simulink model "TST_HLSDem_SelectParameter"  (R2016b)
settings: Solver=FixedStepDiscrete  StartTime=0.0  StopTime=simTime  FixedStep=sampleTime  RelTol=1e-3
values from neighbouring files (symbols this model uses):
  testCase = 1    [initTST_HLSDem_SelectParameter_001.m]    (also in initTST_HLSDem_SelectParameter_002.m = 2; initTST_HLSDem_SelectParameter_003.m = 3; initTST_HLSDem_SelectParameter_004.m = 4; initTST_HLSDem_SelectParameter_005.m = 5)
libraries: simulink x146, UnitTest_Lib x140
(part 4 of 4)

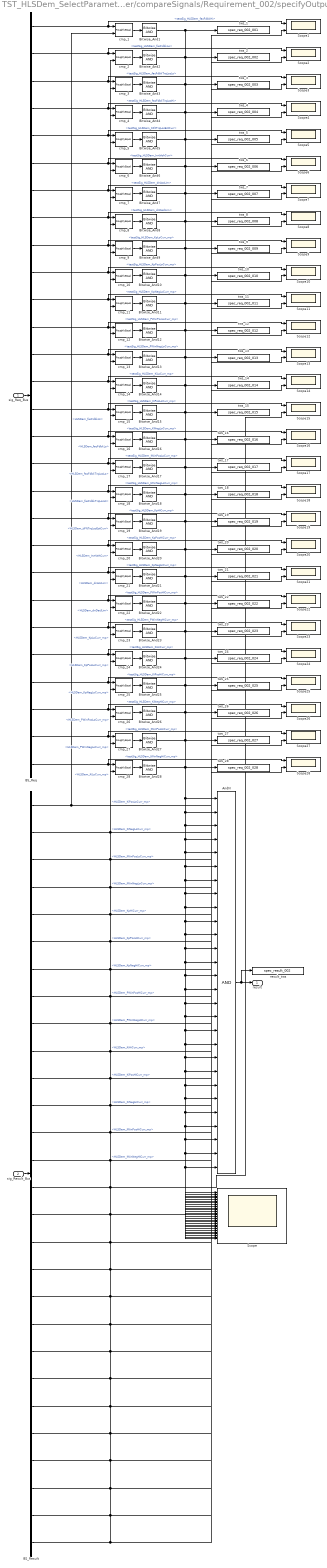
== system TST_HLSDem_SelectParameter/compareSignals/Requirement_002/specifyOutputs ==
  sig_Req_Bus : Inport
  sig_Result_Bus : Inport  Port=2
  AndN : Logic  Inputs=28
  BS_Req : BusSelector  OutputSignals=testSig_HLSDem_facFdbkHi,testSig_HLSDem_facFdbkLo,testSig_HLSDem_facFdbkTrqLosLo,testSig_HLSDem_facFdbkTrqLosHi,testSig_HLSDem_tiFltTrqLosEstCurr,testSig_HLSDem_InrtVehCurr,testSig_HLSDem_dnAccLim,testSig_HLSDem_dnDeclLim,testSig_HLSDem_KpLoCurr_mp,testSig_HLSDem_KpPosLoCurr_mp,testSig_HLSDem_KpNegLoCurr_mp,testSig_HLSDem_PWinPosLoCurr_mp,testSig_HLSDem_PWinNegLoCurr_mp,testSig_HLSDem_KiLoCurr_mp,testSig_HLSDem_KiPosLoCurr_mp,testSig_HLSDem_KiNegLoCurr_mp,testSig_HLSDem_IWinPosLoCurr_mp,testSig_HLSDem_IWinNegLoCurr_mp,testSig_HLSDem_KpHiCurr_mp,testSig_HLSDem_KpPosHiCurr_mp,testSig_HLSDem_KpNegHiCurr_mp,testSig_HLSDem_PWinPosHiCurr_mp,testSig_HLSDem_PWinNegHiCurr_mp,testSig_HLSDem_KiHiCurr_mp,testSig_HLSDem_KiPosHiCurr_mp,testSig_HLSDem_KiNegHiCurr_mp,testSig_HLSDem_IWinPosHiCurr_mp,testSig_HLSDem_IWinNegHiCurr_mp
  BS_Result : BusSelector  OutputSignals=HLSDem_facFdbkHi,HLSDem_facFdbkLo,HLSDem_facFdbkTrqLosLo,HLSDem_facFdbkTrqLosHi,HLSDem_tiFltTrqLosEstCurr,HLSDem_InrtVehCurr,HLSDem_dnAccLim,HLSDem_dnDeclLim,HLSDem_KpLoCurr_mp,HLSDem_KpPosLoCurr_mp,HLSDem_KpNegLoCurr_mp,HLSDem_PWinPosLoCurr_mp,HLSDem_PWinNegLoCurr_mp,HLSDem_KiLoCurr_mp,HLSDem_KiPosLoCurr_mp,HLSDem_KiNegLoCurr_mp,HLSDem_IWinPosLoCurr_mp,HLSDem_IWinNegLoCurr_mp,HLSDem_KpHiCurr_mp,HLSDem_KpPosHiCurr_mp,HLSDem_KpNegHiCurr_mp,HLSDem_PWinPosHiCurr_mp,HLSDem_PWinNegHiCurr_mp,HLSDem_KiHiCurr_mp,HLSDem_KiPosHiCurr_mp,HLSDem_KiNegHiCurr_mp,HLSDem_IWinPosHiCurr_mp,HLSDem_IWinNegHiCurr_mp
  Bitwise_And{1..28} (28 alike) : simulink/Logic and Bit Operations/Bitwise Operator  logicop=AND  UseBitMask=off  BitMask=bin2dec('11011001')  BitMaskRealWorld=Stored Integer
  Scope : Scope  NumInputPorts=28
  Scope{1..28} (28 alike) : Scope  NumInputPorts=2
  cmp_{1..6,9..28} (26 alike) : UnitTest_Lib/RoughlyEqual  slope=0.1
  cmp_7 : UnitTest_Lib/RoughlyEqual  slope=10
  cmp_8 : UnitTest_Lib/RoughlyEqual  slope=10
  result_tws : ToWorkspace  VariableName=spec_result_002
  tws_1 : ToWorkspace  VariableName=spec_req_002_001
  tws_10 : ToWorkspace  VariableName=spec_req_002_010
  tws_11 : ToWorkspace  VariableName=spec_req_002_011
  tws_12 : ToWorkspace  VariableName=spec_req_002_012
  tws_13 : ToWorkspace  VariableName=spec_req_002_013
  tws_14 : ToWorkspace  VariableName=spec_req_002_014
  tws_15 : ToWorkspace  VariableName=spec_req_002_015
  tws_16 : ToWorkspace  VariableName=spec_req_002_016
  tws_17 : ToWorkspace  VariableName=spec_req_002_017
  tws_18 : ToWorkspace  VariableName=spec_req_002_018
  tws_19 : ToWorkspace  VariableName=spec_req_002_019
  tws_2 : ToWorkspace  VariableName=spec_req_002_002
  tws_20 : ToWorkspace  VariableName=spec_req_002_020
  tws_21 : ToWorkspace  VariableName=spec_req_002_021
  tws_22 : ToWorkspace  VariableName=spec_req_002_022
  tws_23 : ToWorkspace  VariableName=spec_req_002_023
  tws_24 : ToWorkspace  VariableName=spec_req_002_024
  tws_25 : ToWorkspace  VariableName=spec_req_002_025
  tws_26 : ToWorkspace  VariableName=spec_req_002_026
  tws_27 : ToWorkspace  VariableName=spec_req_002_027
  tws_28 : ToWorkspace  VariableName=spec_req_002_028
  tws_3 : ToWorkspace  VariableName=spec_req_002_003
  tws_4 : ToWorkspace  VariableName=spec_req_002_004
  tws_5 : ToWorkspace  VariableName=spec_req_002_005
  tws_6 : ToWorkspace  VariableName=spec_req_002_006
  tws_7 : ToWorkspace  VariableName=spec_req_002_007
  tws_8 : ToWorkspace  VariableName=spec_req_002_008
  tws_9 : ToWorkspace  VariableName=spec_req_002_009
  result : Outport
  wires:
  sig_Req_Bus/1 -> BS_Req/1
  sig_Result_Bus/1 -> BS_Result/1
  AndN/1 -> result/1, result_tws/1
  BS_Req/1 -> cmp_1/1, Scope1/1  "<testSig_HLSDem_facFdbkHi>"
  BS_Result/1 -> cmp_1/2, Scope1/2  "<HLSDem_facFdbkHi>"
  cmp_1/1 -> Bitwise_And1/1
  Bitwise_And1/1 -> AndN/1, Scope/1, tws_1/1
  BS_Req/2 -> cmp_2/1, Scope2/1  "<testSig_HLSDem_facFdbkLo>"
  BS_Result/2 -> cmp_2/2, Scope2/2  "<HLSDem_facFdbkLo>"
  cmp_2/1 -> Bitwise_And2/1
  Bitwise_And2/1 -> AndN/2, Scope/2, tws_2/1
  BS_Req/3 -> cmp_3/1, Scope3/1  "<testSig_HLSDem_facFdbkTrqLosLo>"
  BS_Result/3 -> cmp_3/2, Scope3/2  "<HLSDem_facFdbkTrqLosLo>"
  cmp_3/1 -> Bitwise_And3/1
  Bitwise_And3/1 -> AndN/3, Scope/3, tws_3/1
  BS_Req/4 -> cmp_4/1, Scope4/1  "<testSig_HLSDem_facFdbkTrqLosHi>"
  BS_Result/4 -> cmp_4/2, Scope4/2  "<HLSDem_facFdbkTrqLosHi>"
  cmp_4/1 -> Bitwise_And4/1
  Bitwise_And4/1 -> AndN/4, Scope/4, tws_4/1
  BS_Req/5 -> cmp_5/1, Scope5/1  "<testSig_HLSDem_tiFltTrqLosEstCurr>"
  BS_Result/5 -> cmp_5/2, Scope5/2  "<HLSDem_tiFltTrqLosEstCurr>"
  cmp_5/1 -> Bitwise_And5/1
  Bitwise_And5/1 -> AndN/5, Scope/5, tws_5/1
  BS_Req/6 -> cmp_6/1, Scope6/1  "<testSig_HLSDem_InrtVehCurr>"
  BS_Result/6 -> cmp_6/2, Scope6/2  "<HLSDem_InrtVehCurr>"
  cmp_6/1 -> Bitwise_And6/1
  Bitwise_And6/1 -> AndN/6, Scope/6, tws_6/1
  BS_Req/7 -> cmp_7/1, Scope7/1  "<testSig_HLSDem_dnAccLim>"
  BS_Result/7 -> cmp_7/2, Scope7/2  "<HLSDem_dnAccLim>"
  cmp_7/1 -> Bitwise_And7/1
  Bitwise_And7/1 -> AndN/7, Scope/7, tws_7/1
  BS_Req/8 -> cmp_8/1, Scope8/1  "<testSig_HLSDem_dnDeclLim>"
  BS_Result/8 -> cmp_8/2, Scope8/2  "<HLSDem_dnDeclLim>"
  cmp_8/1 -> Bitwise_And8/1
  Bitwise_And8/1 -> AndN/8, Scope/8, tws_8/1
  BS_Req/9 -> cmp_9/1, Scope9/1  "<testSig_HLSDem_KpLoCurr_mp>"
  BS_Result/9 -> cmp_9/2, Scope9/2  "<HLSDem_KpLoCurr_mp>"
  cmp_9/1 -> Bitwise_And9/1
  Bitwise_And9/1 -> AndN/9, Scope/9, tws_9/1
  BS_Req/10 -> cmp_10/1, Scope10/1  "<testSig_HLSDem_KpPosLoCurr_mp>"
  BS_Result/10 -> cmp_10/2, Scope10/2  "<HLSDem_KpPosLoCurr_mp>"
  cmp_10/1 -> Bitwise_And10/1
  Bitwise_And10/1 -> AndN/10, Scope/10, tws_10/1
  BS_Req/11 -> cmp_11/1, Scope11/1  "<testSig_HLSDem_KpNegLoCurr_mp>"
  BS_Result/11 -> cmp_11/2, Scope11/2  "<HLSDem_KpNegLoCurr_mp>"
  cmp_11/1 -> Bitwise_And11/1
  Bitwise_And11/1 -> AndN/11, Scope/11, tws_11/1
  BS_Req/12 -> cmp_12/1, Scope12/1  "<testSig_HLSDem_PWinPosLoCurr_mp>"
  BS_Result/12 -> cmp_12/2, Scope12/2  "<HLSDem_PWinPosLoCurr_mp>"
  cmp_12/1 -> Bitwise_And12/1
  Bitwise_And12/1 -> AndN/12, Scope/12, tws_12/1
  BS_Req/13 -> cmp_13/1, Scope13/1  "<testSig_HLSDem_PWinNegLoCurr_mp>"
  BS_Result/13 -> cmp_13/2, Scope13/2  "<HLSDem_PWinNegLoCurr_mp>"
  cmp_13/1 -> Bitwise_And13/1
  Bitwise_And13/1 -> AndN/13, Scope/13, tws_13/1
  BS_Req/14 -> cmp_14/1, Scope14/1  "<testSig_HLSDem_KiLoCurr_mp>"
  BS_Result/14 -> cmp_14/2, Scope14/2  "<HLSDem_KiLoCurr_mp>"
  cmp_14/1 -> Bitwise_And14/1
  Bitwise_And14/1 -> AndN/14, Scope/14, tws_14/1
  BS_Req/15 -> cmp_15/1, Scope15/1  "<testSig_HLSDem_KiPosLoCurr_mp>"
  BS_Result/15 -> cmp_15/2, Scope15/2  "<HLSDem_KiPosLoCurr_mp>"
  cmp_15/1 -> Bitwise_And15/1
  Bitwise_And15/1 -> AndN/15, Scope/15, tws_15/1
  BS_Req/16 -> cmp_16/1, Scope16/1  "<testSig_HLSDem_KiNegLoCurr_mp>"
  BS_Result/16 -> cmp_16/2, Scope16/2  "<HLSDem_KiNegLoCurr_mp>"
  cmp_16/1 -> Bitwise_And16/1
  Bitwise_And16/1 -> AndN/16, Scope/16, tws_16/1
  BS_Req/17 -> cmp_17/1, Scope17/1  "<testSig_HLSDem_IWinPosLoCurr_mp>"
  BS_Result/17 -> cmp_17/2, Scope17/2  "<HLSDem_IWinPosLoCurr_mp>"
  cmp_17/1 -> Bitwise_And17/1
  Bitwise_And17/1 -> AndN/17, Scope/17, tws_17/1
  BS_Req/18 -> cmp_18/1, Scope18/1  "<testSig_HLSDem_IWinNegLoCurr_mp>"
  BS_Result/18 -> cmp_18/2, Scope18/2  "<HLSDem_IWinNegLoCurr_mp>"
  cmp_18/1 -> Bitwise_And18/1
  Bitwise_And18/1 -> AndN/18, Scope/18, tws_18/1
  BS_Req/19 -> cmp_19/1, Scope19/1  "<testSig_HLSDem_KpHiCurr_mp>"
  BS_Result/19 -> cmp_19/2, Scope19/2  "<HLSDem_KpHiCurr_mp>"
  cmp_19/1 -> Bitwise_And19/1
  Bitwise_And19/1 -> AndN/19, Scope/19, tws_19/1
  BS_Req/20 -> cmp_20/1, Scope20/1  "<testSig_HLSDem_KpPosHiCurr_mp>"
  BS_Result/20 -> cmp_20/2, Scope20/2  "<HLSDem_KpPosHiCurr_mp>"
  cmp_20/1 -> Bitwise_And20/1
  Bitwise_And20/1 -> AndN/20, Scope/20, tws_20/1
  BS_Req/21 -> cmp_21/1, Scope21/1  "<testSig_HLSDem_KpNegHiCurr_mp>"
  BS_Result/21 -> cmp_21/2, Scope21/2  "<HLSDem_KpNegHiCurr_mp>"
  cmp_21/1 -> Bitwise_And21/1
  Bitwise_And21/1 -> AndN/21, Scope/21, tws_21/1
  BS_Req/22 -> cmp_22/1, Scope22/1  "<testSig_HLSDem_PWinPosHiCurr_mp>"
  BS_Result/22 -> cmp_22/2, Scope22/2  "<HLSDem_PWinPosHiCurr_mp>"
  cmp_22/1 -> Bitwise_And22/1
  Bitwise_And22/1 -> AndN/22, Scope/22, tws_22/1
  BS_Req/23 -> cmp_23/1, Scope23/1  "<testSig_HLSDem_PWinNegHiCurr_mp>"
  BS_Result/23 -> cmp_23/2, Scope23/2  "<HLSDem_PWinNegHiCurr_mp>"
  cmp_23/1 -> Bitwise_And23/1
  Bitwise_And23/1 -> AndN/23, Scope/23, tws_23/1
  BS_Req/24 -> cmp_24/1, Scope24/1  "<testSig_HLSDem_KiHiCurr_mp>"
  BS_Result/24 -> cmp_24/2, Scope24/2  "<HLSDem_KiHiCurr_mp>"
  cmp_24/1 -> Bitwise_And24/1
  Bitwise_And24/1 -> AndN/24, Scope/24, tws_24/1
  BS_Req/25 -> cmp_25/1, Scope25/1  "<testSig_HLSDem_KiPosHiCurr_mp>"
  BS_Result/25 -> cmp_25/2, Scope25/2  "<HLSDem_KiPosHiCurr_mp>"
  cmp_25/1 -> Bitwise_And25/1
  Bitwise_And25/1 -> AndN/25, Scope/25, tws_25/1
  BS_Req/26 -> cmp_26/1, Scope26/1  "<testSig_HLSDem_KiNegHiCurr_mp>"
  BS_Result/26 -> cmp_26/2, Scope26/2  "<HLSDem_KiNegHiCurr_mp>"
  cmp_26/1 -> Bitwise_And26/1
  Bitwise_And26/1 -> AndN/26, Scope/26, tws_26/1
  BS_Req/27 -> cmp_27/1, Scope27/1  "<testSig_HLSDem_IWinPosHiCurr_mp>"
  BS_Result/27 -> cmp_27/2, Scope27/2  "<HLSDem_IWinPosHiCurr_mp>"
  cmp_27/1 -> Bitwise_And27/1
  Bitwise_And27/1 -> AndN/27, Scope/27, tws_27/1
  BS_Req/28 -> cmp_28/1, Scope28/1  "<testSig_HLSDem_IWinNegHiCurr_mp>"
  BS_Result/28 -> cmp_28/2, Scope28/2  "<HLSDem_IWinNegHiCurr_mp>"
  cmp_28/1 -> Bitwise_And28/1
  Bitwise_And28/1 -> AndN/28, Scope/28, tws_28/1

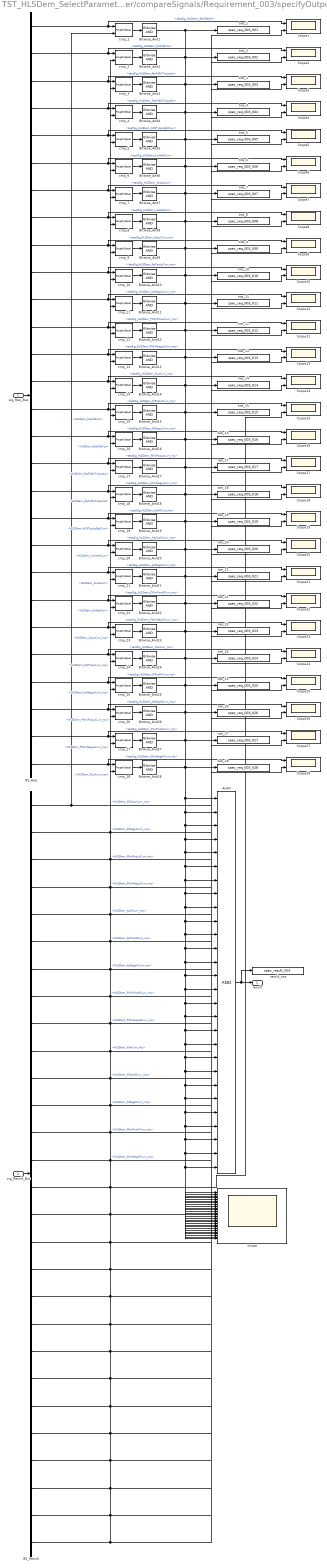
== system TST_HLSDem_SelectParameter/compareSignals/Requirement_003/specifyOutputs ==
  sig_Req_Bus : Inport
  sig_Result_Bus : Inport  Port=2
  AndN : Logic  Inputs=28
  BS_Req : BusSelector  OutputSignals=testSig_HLSDem_facFdbkHi,testSig_HLSDem_facFdbkLo,testSig_HLSDem_facFdbkTrqLosLo,testSig_HLSDem_facFdbkTrqLosHi,testSig_HLSDem_tiFltTrqLosEstCurr,testSig_HLSDem_InrtVehCurr,testSig_HLSDem_dnAccLim,testSig_HLSDem_dnDeclLim,testSig_HLSDem_KpLoCurr_mp,testSig_HLSDem_KpPosLoCurr_mp,testSig_HLSDem_KpNegLoCurr_mp,testSig_HLSDem_PWinPosLoCurr_mp,testSig_HLSDem_PWinNegLoCurr_mp,testSig_HLSDem_KiLoCurr_mp,testSig_HLSDem_KiPosLoCurr_mp,testSig_HLSDem_KiNegLoCurr_mp,testSig_HLSDem_IWinPosLoCurr_mp,testSig_HLSDem_IWinNegLoCurr_mp,testSig_HLSDem_KpHiCurr_mp,testSig_HLSDem_KpPosHiCurr_mp,testSig_HLSDem_KpNegHiCurr_mp,testSig_HLSDem_PWinPosHiCurr_mp,testSig_HLSDem_PWinNegHiCurr_mp,testSig_HLSDem_KiHiCurr_mp,testSig_HLSDem_KiPosHiCurr_mp,testSig_HLSDem_KiNegHiCurr_mp,testSig_HLSDem_IWinPosHiCurr_mp,testSig_HLSDem_IWinNegHiCurr_mp
  BS_Result : BusSelector  OutputSignals=HLSDem_facFdbkHi,HLSDem_facFdbkLo,HLSDem_facFdbkTrqLosLo,HLSDem_facFdbkTrqLosHi,HLSDem_tiFltTrqLosEstCurr,HLSDem_InrtVehCurr,HLSDem_dnAccLim,HLSDem_dnDeclLim,HLSDem_KpLoCurr_mp,HLSDem_KpPosLoCurr_mp,HLSDem_KpNegLoCurr_mp,HLSDem_PWinPosLoCurr_mp,HLSDem_PWinNegLoCurr_mp,HLSDem_KiLoCurr_mp,HLSDem_KiPosLoCurr_mp,HLSDem_KiNegLoCurr_mp,HLSDem_IWinPosLoCurr_mp,HLSDem_IWinNegLoCurr_mp,HLSDem_KpHiCurr_mp,HLSDem_KpPosHiCurr_mp,HLSDem_KpNegHiCurr_mp,HLSDem_PWinPosHiCurr_mp,HLSDem_PWinNegHiCurr_mp,HLSDem_KiHiCurr_mp,HLSDem_KiPosHiCurr_mp,HLSDem_KiNegHiCurr_mp,HLSDem_IWinPosHiCurr_mp,HLSDem_IWinNegHiCurr_mp
  Bitwise_And{1..28} (28 alike) : simulink/Logic and Bit Operations/Bitwise Operator  logicop=AND  UseBitMask=off  BitMask=bin2dec('11011001')  BitMaskRealWorld=Stored Integer
  Scope : Scope  NumInputPorts=28
  Scope{1..28} (28 alike) : Scope  NumInputPorts=2
  cmp_{1..6,9..28} (26 alike) : UnitTest_Lib/RoughlyEqual  slope=0.1
  cmp_7 : UnitTest_Lib/RoughlyEqual  slope=1
  cmp_8 : UnitTest_Lib/RoughlyEqual  slope=1
  result_tws : ToWorkspace  VariableName=spec_result_003
  tws_1 : ToWorkspace  VariableName=spec_req_003_001
  tws_10 : ToWorkspace  VariableName=spec_req_003_010
  tws_11 : ToWorkspace  VariableName=spec_req_003_011
  tws_12 : ToWorkspace  VariableName=spec_req_003_012
  tws_13 : ToWorkspace  VariableName=spec_req_003_013
  tws_14 : ToWorkspace  VariableName=spec_req_003_014
  tws_15 : ToWorkspace  VariableName=spec_req_003_015
  tws_16 : ToWorkspace  VariableName=spec_req_003_016
  tws_17 : ToWorkspace  VariableName=spec_req_003_017
  tws_18 : ToWorkspace  VariableName=spec_req_003_018
  tws_19 : ToWorkspace  VariableName=spec_req_003_019
  tws_2 : ToWorkspace  VariableName=spec_req_003_002
  tws_20 : ToWorkspace  VariableName=spec_req_003_020
  tws_21 : ToWorkspace  VariableName=spec_req_003_021
  tws_22 : ToWorkspace  VariableName=spec_req_003_022
  tws_23 : ToWorkspace  VariableName=spec_req_003_023
  tws_24 : ToWorkspace  VariableName=spec_req_003_024
  tws_25 : ToWorkspace  VariableName=spec_req_003_025
  tws_26 : ToWorkspace  VariableName=spec_req_003_026
  tws_27 : ToWorkspace  VariableName=spec_req_003_027
  tws_28 : ToWorkspace  VariableName=spec_req_003_028
  tws_3 : ToWorkspace  VariableName=spec_req_003_003
  tws_4 : ToWorkspace  VariableName=spec_req_003_004
  tws_5 : ToWorkspace  VariableName=spec_req_003_005
  tws_6 : ToWorkspace  VariableName=spec_req_003_006
  tws_7 : ToWorkspace  VariableName=spec_req_003_007
  tws_8 : ToWorkspace  VariableName=spec_req_003_008
  tws_9 : ToWorkspace  VariableName=spec_req_003_009
  result : Outport
  wires:
  sig_Req_Bus/1 -> BS_Req/1
  sig_Result_Bus/1 -> BS_Result/1
  AndN/1 -> result/1, result_tws/1
  BS_Req/1 -> cmp_1/1, Scope1/1  "<testSig_HLSDem_facFdbkHi>"
  BS_Result/1 -> cmp_1/2, Scope1/2  "<HLSDem_facFdbkHi>"
  cmp_1/1 -> Bitwise_And1/1
  Bitwise_And1/1 -> AndN/1, Scope/1, tws_1/1
  BS_Req/2 -> cmp_2/1, Scope2/1  "<testSig_HLSDem_facFdbkLo>"
  BS_Result/2 -> cmp_2/2, Scope2/2  "<HLSDem_facFdbkLo>"
  cmp_2/1 -> Bitwise_And2/1
  Bitwise_And2/1 -> AndN/2, Scope/2, tws_2/1
  BS_Req/3 -> cmp_3/1, Scope3/1  "<testSig_HLSDem_facFdbkTrqLosLo>"
  BS_Result/3 -> cmp_3/2, Scope3/2  "<HLSDem_facFdbkTrqLosLo>"
  cmp_3/1 -> Bitwise_And3/1
  Bitwise_And3/1 -> AndN/3, Scope/3, tws_3/1
  BS_Req/4 -> cmp_4/1, Scope4/1  "<testSig_HLSDem_facFdbkTrqLosHi>"
  BS_Result/4 -> cmp_4/2, Scope4/2  "<HLSDem_facFdbkTrqLosHi>"
  cmp_4/1 -> Bitwise_And4/1
  Bitwise_And4/1 -> AndN/4, Scope/4, tws_4/1
  BS_Req/5 -> cmp_5/1, Scope5/1  "<testSig_HLSDem_tiFltTrqLosEstCurr>"
  BS_Result/5 -> cmp_5/2, Scope5/2  "<HLSDem_tiFltTrqLosEstCurr>"
  cmp_5/1 -> Bitwise_And5/1
  Bitwise_And5/1 -> AndN/5, Scope/5, tws_5/1
  BS_Req/6 -> cmp_6/1, Scope6/1  "<testSig_HLSDem_InrtVehCurr>"
  BS_Result/6 -> cmp_6/2, Scope6/2  "<HLSDem_InrtVehCurr>"
  cmp_6/1 -> Bitwise_And6/1
  Bitwise_And6/1 -> AndN/6, Scope/6, tws_6/1
  BS_Req/7 -> cmp_7/1, Scope7/1  "<testSig_HLSDem_dnAccLim>"
  BS_Result/7 -> cmp_7/2, Scope7/2  "<HLSDem_dnAccLim>"
  cmp_7/1 -> Bitwise_And7/1
  Bitwise_And7/1 -> AndN/7, Scope/7, tws_7/1
  BS_Req/8 -> cmp_8/1, Scope8/1  "<testSig_HLSDem_dnDeclLim>"
  BS_Result/8 -> cmp_8/2, Scope8/2  "<HLSDem_dnDeclLim>"
  cmp_8/1 -> Bitwise_And8/1
  Bitwise_And8/1 -> AndN/8, Scope/8, tws_8/1
  BS_Req/9 -> cmp_9/1, Scope9/1  "<testSig_HLSDem_KpLoCurr_mp>"
  BS_Result/9 -> cmp_9/2, Scope9/2  "<HLSDem_KpLoCurr_mp>"
  cmp_9/1 -> Bitwise_And9/1
  Bitwise_And9/1 -> AndN/9, Scope/9, tws_9/1
  BS_Req/10 -> cmp_10/1, Scope10/1  "<testSig_HLSDem_KpPosLoCurr_mp>"
  BS_Result/10 -> cmp_10/2, Scope10/2  "<HLSDem_KpPosLoCurr_mp>"
  cmp_10/1 -> Bitwise_And10/1
  Bitwise_And10/1 -> AndN/10, Scope/10, tws_10/1
  BS_Req/11 -> cmp_11/1, Scope11/1  "<testSig_HLSDem_KpNegLoCurr_mp>"
  BS_Result/11 -> cmp_11/2, Scope11/2  "<HLSDem_KpNegLoCurr_mp>"
  cmp_11/1 -> Bitwise_And11/1
  Bitwise_And11/1 -> AndN/11, Scope/11, tws_11/1
  BS_Req/12 -> cmp_12/1, Scope12/1  "<testSig_HLSDem_PWinPosLoCurr_mp>"
  BS_Result/12 -> cmp_12/2, Scope12/2  "<HLSDem_PWinPosLoCurr_mp>"
  cmp_12/1 -> Bitwise_And12/1
  Bitwise_And12/1 -> AndN/12, Scope/12, tws_12/1
  BS_Req/13 -> cmp_13/1, Scope13/1  "<testSig_HLSDem_PWinNegLoCurr_mp>"
  BS_Result/13 -> cmp_13/2, Scope13/2  "<HLSDem_PWinNegLoCurr_mp>"
  cmp_13/1 -> Bitwise_And13/1
  Bitwise_And13/1 -> AndN/13, Scope/13, tws_13/1
  BS_Req/14 -> cmp_14/1, Scope14/1  "<testSig_HLSDem_KiLoCurr_mp>"
  BS_Result/14 -> cmp_14/2, Scope14/2  "<HLSDem_KiLoCurr_mp>"
  cmp_14/1 -> Bitwise_And14/1
  Bitwise_And14/1 -> AndN/14, Scope/14, tws_14/1
  BS_Req/15 -> cmp_15/1, Scope15/1  "<testSig_HLSDem_KiPosLoCurr_mp>"
  BS_Result/15 -> cmp_15/2, Scope15/2  "<HLSDem_KiPosLoCurr_mp>"
  cmp_15/1 -> Bitwise_And15/1
  Bitwise_And15/1 -> AndN/15, Scope/15, tws_15/1
  BS_Req/16 -> cmp_16/1, Scope16/1  "<testSig_HLSDem_KiNegLoCurr_mp>"
  BS_Result/16 -> cmp_16/2, Scope16/2  "<HLSDem_KiNegLoCurr_mp>"
  cmp_16/1 -> Bitwise_And16/1
  Bitwise_And16/1 -> AndN/16, Scope/16, tws_16/1
  BS_Req/17 -> cmp_17/1, Scope17/1  "<testSig_HLSDem_IWinPosLoCurr_mp>"
  BS_Result/17 -> cmp_17/2, Scope17/2  "<HLSDem_IWinPosLoCurr_mp>"
  cmp_17/1 -> Bitwise_And17/1
  Bitwise_And17/1 -> AndN/17, Scope/17, tws_17/1
  BS_Req/18 -> cmp_18/1, Scope18/1  "<testSig_HLSDem_IWinNegLoCurr_mp>"
  BS_Result/18 -> cmp_18/2, Scope18/2  "<HLSDem_IWinNegLoCurr_mp>"
  cmp_18/1 -> Bitwise_And18/1
  Bitwise_And18/1 -> AndN/18, Scope/18, tws_18/1
  BS_Req/19 -> cmp_19/1, Scope19/1  "<testSig_HLSDem_KpHiCurr_mp>"
  BS_Result/19 -> cmp_19/2, Scope19/2  "<HLSDem_KpHiCurr_mp>"
  cmp_19/1 -> Bitwise_And19/1
  Bitwise_And19/1 -> AndN/19, Scope/19, tws_19/1
  BS_Req/20 -> cmp_20/1, Scope20/1  "<testSig_HLSDem_KpPosHiCurr_mp>"
  BS_Result/20 -> cmp_20/2, Scope20/2  "<HLSDem_KpPosHiCurr_mp>"
  cmp_20/1 -> Bitwise_And20/1
  Bitwise_And20/1 -> AndN/20, Scope/20, tws_20/1
  BS_Req/21 -> cmp_21/1, Scope21/1  "<testSig_HLSDem_KpNegHiCurr_mp>"
  BS_Result/21 -> cmp_21/2, Scope21/2  "<HLSDem_KpNegHiCurr_mp>"
  cmp_21/1 -> Bitwise_And21/1
  Bitwise_And21/1 -> AndN/21, Scope/21, tws_21/1
  BS_Req/22 -> cmp_22/1, Scope22/1  "<testSig_HLSDem_PWinPosHiCurr_mp>"
  BS_Result/22 -> cmp_22/2, Scope22/2  "<HLSDem_PWinPosHiCurr_mp>"
  cmp_22/1 -> Bitwise_And22/1
  Bitwise_And22/1 -> AndN/22, Scope/22, tws_22/1
  BS_Req/23 -> cmp_23/1, Scope23/1  "<testSig_HLSDem_PWinNegHiCurr_mp>"
  BS_Result/23 -> cmp_23/2, Scope23/2  "<HLSDem_PWinNegHiCurr_mp>"
  cmp_23/1 -> Bitwise_And23/1
  Bitwise_And23/1 -> AndN/23, Scope/23, tws_23/1
  BS_Req/24 -> cmp_24/1, Scope24/1  "<testSig_HLSDem_KiHiCurr_mp>"
  BS_Result/24 -> cmp_24/2, Scope24/2  "<HLSDem_KiHiCurr_mp>"
  cmp_24/1 -> Bitwise_And24/1
  Bitwise_And24/1 -> AndN/24, Scope/24, tws_24/1
  BS_Req/25 -> cmp_25/1, Scope25/1  "<testSig_HLSDem_KiPosHiCurr_mp>"
  BS_Result/25 -> cmp_25/2, Scope25/2  "<HLSDem_KiPosHiCurr_mp>"
  cmp_25/1 -> Bitwise_And25/1
  Bitwise_And25/1 -> AndN/25, Scope/25, tws_25/1
  BS_Req/26 -> cmp_26/1, Scope26/1  "<testSig_HLSDem_KiNegHiCurr_mp>"
  BS_Result/26 -> cmp_26/2, Scope26/2  "<HLSDem_KiNegHiCurr_mp>"
  cmp_26/1 -> Bitwise_And26/1
  Bitwise_And26/1 -> AndN/26, Scope/26, tws_26/1
  BS_Req/27 -> cmp_27/1, Scope27/1  "<testSig_HLSDem_IWinPosHiCurr_mp>"
  BS_Result/27 -> cmp_27/2, Scope27/2  "<HLSDem_IWinPosHiCurr_mp>"
  cmp_27/1 -> Bitwise_And27/1
  Bitwise_And27/1 -> AndN/27, Scope/27, tws_27/1
  BS_Req/28 -> cmp_28/1, Scope28/1  "<testSig_HLSDem_IWinNegHiCurr_mp>"
  BS_Result/28 -> cmp_28/2, Scope28/2  "<HLSDem_IWinNegHiCurr_mp>"
  cmp_28/1 -> Bitwise_And28/1
  Bitwise_And28/1 -> AndN/28, Scope/28, tws_28/1

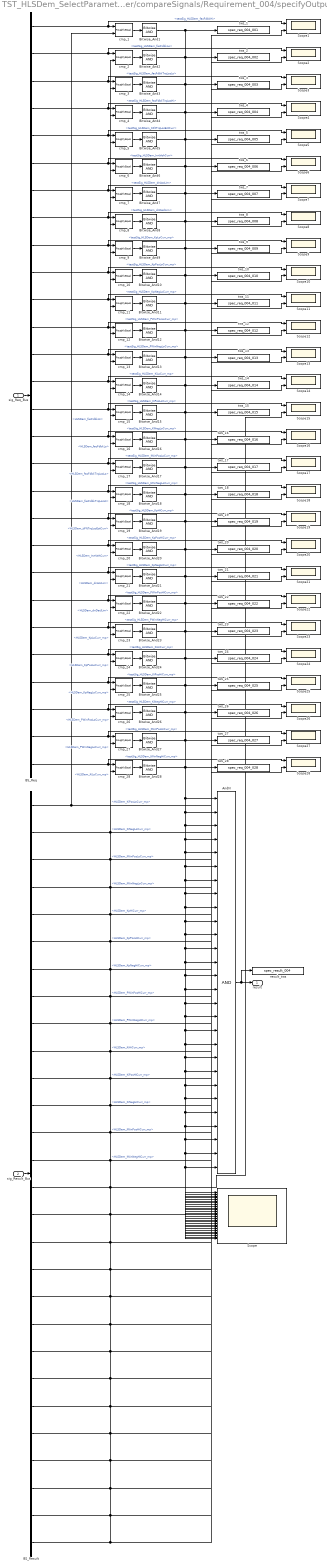
== system TST_HLSDem_SelectParameter/compareSignals/Requirement_004/specifyOutputs ==
  sig_Req_Bus : Inport
  sig_Result_Bus : Inport  Port=2
  AndN : Logic  Inputs=28
  BS_Req : BusSelector  OutputSignals=testSig_HLSDem_facFdbkHi,testSig_HLSDem_facFdbkLo,testSig_HLSDem_facFdbkTrqLosLo,testSig_HLSDem_facFdbkTrqLosHi,testSig_HLSDem_tiFltTrqLosEstCurr,testSig_HLSDem_InrtVehCurr,testSig_HLSDem_dnAccLim,testSig_HLSDem_dnDeclLim,testSig_HLSDem_KpLoCurr_mp,testSig_HLSDem_KpPosLoCurr_mp,testSig_HLSDem_KpNegLoCurr_mp,testSig_HLSDem_PWinPosLoCurr_mp,testSig_HLSDem_PWinNegLoCurr_mp,testSig_HLSDem_KiLoCurr_mp,testSig_HLSDem_KiPosLoCurr_mp,testSig_HLSDem_KiNegLoCurr_mp,testSig_HLSDem_IWinPosLoCurr_mp,testSig_HLSDem_IWinNegLoCurr_mp,testSig_HLSDem_KpHiCurr_mp,testSig_HLSDem_KpPosHiCurr_mp,testSig_HLSDem_KpNegHiCurr_mp,testSig_HLSDem_PWinPosHiCurr_mp,testSig_HLSDem_PWinNegHiCurr_mp,testSig_HLSDem_KiHiCurr_mp,testSig_HLSDem_KiPosHiCurr_mp,testSig_HLSDem_KiNegHiCurr_mp,testSig_HLSDem_IWinPosHiCurr_mp,testSig_HLSDem_IWinNegHiCurr_mp
  BS_Result : BusSelector  OutputSignals=HLSDem_facFdbkHi,HLSDem_facFdbkLo,HLSDem_facFdbkTrqLosLo,HLSDem_facFdbkTrqLosHi,HLSDem_tiFltTrqLosEstCurr,HLSDem_InrtVehCurr,HLSDem_dnAccLim,HLSDem_dnDeclLim,HLSDem_KpLoCurr_mp,HLSDem_KpPosLoCurr_mp,HLSDem_KpNegLoCurr_mp,HLSDem_PWinPosLoCurr_mp,HLSDem_PWinNegLoCurr_mp,HLSDem_KiLoCurr_mp,HLSDem_KiPosLoCurr_mp,HLSDem_KiNegLoCurr_mp,HLSDem_IWinPosLoCurr_mp,HLSDem_IWinNegLoCurr_mp,HLSDem_KpHiCurr_mp,HLSDem_KpPosHiCurr_mp,HLSDem_KpNegHiCurr_mp,HLSDem_PWinPosHiCurr_mp,HLSDem_PWinNegHiCurr_mp,HLSDem_KiHiCurr_mp,HLSDem_KiPosHiCurr_mp,HLSDem_KiNegHiCurr_mp,HLSDem_IWinPosHiCurr_mp,HLSDem_IWinNegHiCurr_mp
  Bitwise_And{1..28} (28 alike) : simulink/Logic and Bit Operations/Bitwise Operator  logicop=AND  UseBitMask=off  BitMask=bin2dec('11011001')  BitMaskRealWorld=Stored Integer
  Scope : Scope  NumInputPorts=28
  Scope{1..28} (28 alike) : Scope  NumInputPorts=2
  cmp_{1..6,9..28} (26 alike) : UnitTest_Lib/RoughlyEqual  slope=0.1
  cmp_7 : UnitTest_Lib/RoughlyEqual  slope=1
  cmp_8 : UnitTest_Lib/RoughlyEqual  slope=1
  result_tws : ToWorkspace  VariableName=spec_result_004
  tws_1 : ToWorkspace  VariableName=spec_req_004_001
  tws_10 : ToWorkspace  VariableName=spec_req_004_010
  tws_11 : ToWorkspace  VariableName=spec_req_004_011
  tws_12 : ToWorkspace  VariableName=spec_req_004_012
  tws_13 : ToWorkspace  VariableName=spec_req_004_013
  tws_14 : ToWorkspace  VariableName=spec_req_004_014
  tws_15 : ToWorkspace  VariableName=spec_req_004_015
  tws_16 : ToWorkspace  VariableName=spec_req_004_016
  tws_17 : ToWorkspace  VariableName=spec_req_004_017
  tws_18 : ToWorkspace  VariableName=spec_req_004_018
  tws_19 : ToWorkspace  VariableName=spec_req_004_019
  tws_2 : ToWorkspace  VariableName=spec_req_004_002
  tws_20 : ToWorkspace  VariableName=spec_req_004_020
  tws_21 : ToWorkspace  VariableName=spec_req_004_021
  tws_22 : ToWorkspace  VariableName=spec_req_004_022
  tws_23 : ToWorkspace  VariableName=spec_req_004_023
  tws_24 : ToWorkspace  VariableName=spec_req_004_024
  tws_25 : ToWorkspace  VariableName=spec_req_004_025
  tws_26 : ToWorkspace  VariableName=spec_req_004_026
  tws_27 : ToWorkspace  VariableName=spec_req_004_027
  tws_28 : ToWorkspace  VariableName=spec_req_004_028
  tws_3 : ToWorkspace  VariableName=spec_req_004_003
  tws_4 : ToWorkspace  VariableName=spec_req_004_004
  tws_5 : ToWorkspace  VariableName=spec_req_004_005
  tws_6 : ToWorkspace  VariableName=spec_req_004_006
  tws_7 : ToWorkspace  VariableName=spec_req_004_007
  tws_8 : ToWorkspace  VariableName=spec_req_004_008
  tws_9 : ToWorkspace  VariableName=spec_req_004_009
  result : Outport
  wires:
  sig_Req_Bus/1 -> BS_Req/1
  sig_Result_Bus/1 -> BS_Result/1
  AndN/1 -> result/1, result_tws/1
  BS_Req/1 -> cmp_1/1, Scope1/1  "<testSig_HLSDem_facFdbkHi>"
  BS_Result/1 -> cmp_1/2, Scope1/2  "<HLSDem_facFdbkHi>"
  cmp_1/1 -> Bitwise_And1/1
  Bitwise_And1/1 -> AndN/1, Scope/1, tws_1/1
  BS_Req/2 -> cmp_2/1, Scope2/1  "<testSig_HLSDem_facFdbkLo>"
  BS_Result/2 -> cmp_2/2, Scope2/2  "<HLSDem_facFdbkLo>"
  cmp_2/1 -> Bitwise_And2/1
  Bitwise_And2/1 -> AndN/2, Scope/2, tws_2/1
  BS_Req/3 -> cmp_3/1, Scope3/1  "<testSig_HLSDem_facFdbkTrqLosLo>"
  BS_Result/3 -> cmp_3/2, Scope3/2  "<HLSDem_facFdbkTrqLosLo>"
  cmp_3/1 -> Bitwise_And3/1
  Bitwise_And3/1 -> AndN/3, Scope/3, tws_3/1
  BS_Req/4 -> cmp_4/1, Scope4/1  "<testSig_HLSDem_facFdbkTrqLosHi>"
  BS_Result/4 -> cmp_4/2, Scope4/2  "<HLSDem_facFdbkTrqLosHi>"
  cmp_4/1 -> Bitwise_And4/1
  Bitwise_And4/1 -> AndN/4, Scope/4, tws_4/1
  BS_Req/5 -> cmp_5/1, Scope5/1  "<testSig_HLSDem_tiFltTrqLosEstCurr>"
  BS_Result/5 -> cmp_5/2, Scope5/2  "<HLSDem_tiFltTrqLosEstCurr>"
  cmp_5/1 -> Bitwise_And5/1
  Bitwise_And5/1 -> AndN/5, Scope/5, tws_5/1
  BS_Req/6 -> cmp_6/1, Scope6/1  "<testSig_HLSDem_InrtVehCurr>"
  BS_Result/6 -> cmp_6/2, Scope6/2  "<HLSDem_InrtVehCurr>"
  cmp_6/1 -> Bitwise_And6/1
  Bitwise_And6/1 -> AndN/6, Scope/6, tws_6/1
  BS_Req/7 -> cmp_7/1, Scope7/1  "<testSig_HLSDem_dnAccLim>"
  BS_Result/7 -> cmp_7/2, Scope7/2  "<HLSDem_dnAccLim>"
  cmp_7/1 -> Bitwise_And7/1
  Bitwise_And7/1 -> AndN/7, Scope/7, tws_7/1
  BS_Req/8 -> cmp_8/1, Scope8/1  "<testSig_HLSDem_dnDeclLim>"
  BS_Result/8 -> cmp_8/2, Scope8/2  "<HLSDem_dnDeclLim>"
  cmp_8/1 -> Bitwise_And8/1
  Bitwise_And8/1 -> AndN/8, Scope/8, tws_8/1
  BS_Req/9 -> cmp_9/1, Scope9/1  "<testSig_HLSDem_KpLoCurr_mp>"
  BS_Result/9 -> cmp_9/2, Scope9/2  "<HLSDem_KpLoCurr_mp>"
  cmp_9/1 -> Bitwise_And9/1
  Bitwise_And9/1 -> AndN/9, Scope/9, tws_9/1
  BS_Req/10 -> cmp_10/1, Scope10/1  "<testSig_HLSDem_KpPosLoCurr_mp>"
  BS_Result/10 -> cmp_10/2, Scope10/2  "<HLSDem_KpPosLoCurr_mp>"
  cmp_10/1 -> Bitwise_And10/1
  Bitwise_And10/1 -> AndN/10, Scope/10, tws_10/1
  BS_Req/11 -> cmp_11/1, Scope11/1  "<testSig_HLSDem_KpNegLoCurr_mp>"
  BS_Result/11 -> cmp_11/2, Scope11/2  "<HLSDem_KpNegLoCurr_mp>"
  cmp_11/1 -> Bitwise_And11/1
  Bitwise_And11/1 -> AndN/11, Scope/11, tws_11/1
  BS_Req/12 -> cmp_12/1, Scope12/1  "<testSig_HLSDem_PWinPosLoCurr_mp>"
  BS_Result/12 -> cmp_12/2, Scope12/2  "<HLSDem_PWinPosLoCurr_mp>"
  cmp_12/1 -> Bitwise_And12/1
  Bitwise_And12/1 -> AndN/12, Scope/12, tws_12/1
  BS_Req/13 -> cmp_13/1, Scope13/1  "<testSig_HLSDem_PWinNegLoCurr_mp>"
  BS_Result/13 -> cmp_13/2, Scope13/2  "<HLSDem_PWinNegLoCurr_mp>"
  cmp_13/1 -> Bitwise_And13/1
  Bitwise_And13/1 -> AndN/13, Scope/13, tws_13/1
  BS_Req/14 -> cmp_14/1, Scope14/1  "<testSig_HLSDem_KiLoCurr_mp>"
  BS_Result/14 -> cmp_14/2, Scope14/2  "<HLSDem_KiLoCurr_mp>"
  cmp_14/1 -> Bitwise_And14/1
  Bitwise_And14/1 -> AndN/14, Scope/14, tws_14/1
  BS_Req/15 -> cmp_15/1, Scope15/1  "<testSig_HLSDem_KiPosLoCurr_mp>"
  BS_Result/15 -> cmp_15/2, Scope15/2  "<HLSDem_KiPosLoCurr_mp>"
  cmp_15/1 -> Bitwise_And15/1
  Bitwise_And15/1 -> AndN/15, Scope/15, tws_15/1
  BS_Req/16 -> cmp_16/1, Scope16/1  "<testSig_HLSDem_KiNegLoCurr_mp>"
  BS_Result/16 -> cmp_16/2, Scope16/2  "<HLSDem_KiNegLoCurr_mp>"
  cmp_16/1 -> Bitwise_And16/1
  Bitwise_And16/1 -> AndN/16, Scope/16, tws_16/1
  BS_Req/17 -> cmp_17/1, Scope17/1  "<testSig_HLSDem_IWinPosLoCurr_mp>"
  BS_Result/17 -> cmp_17/2, Scope17/2  "<HLSDem_IWinPosLoCurr_mp>"
  cmp_17/1 -> Bitwise_And17/1
  Bitwise_And17/1 -> AndN/17, Scope/17, tws_17/1
  BS_Req/18 -> cmp_18/1, Scope18/1  "<testSig_HLSDem_IWinNegLoCurr_mp>"
  BS_Result/18 -> cmp_18/2, Scope18/2  "<HLSDem_IWinNegLoCurr_mp>"
  cmp_18/1 -> Bitwise_And18/1
  Bitwise_And18/1 -> AndN/18, Scope/18, tws_18/1
  BS_Req/19 -> cmp_19/1, Scope19/1  "<testSig_HLSDem_KpHiCurr_mp>"
  BS_Result/19 -> cmp_19/2, Scope19/2  "<HLSDem_KpHiCurr_mp>"
  cmp_19/1 -> Bitwise_And19/1
  Bitwise_And19/1 -> AndN/19, Scope/19, tws_19/1
  BS_Req/20 -> cmp_20/1, Scope20/1  "<testSig_HLSDem_KpPosHiCurr_mp>"
  BS_Result/20 -> cmp_20/2, Scope20/2  "<HLSDem_KpPosHiCurr_mp>"
  cmp_20/1 -> Bitwise_And20/1
  Bitwise_And20/1 -> AndN/20, Scope/20, tws_20/1
  BS_Req/21 -> cmp_21/1, Scope21/1  "<testSig_HLSDem_KpNegHiCurr_mp>"
  BS_Result/21 -> cmp_21/2, Scope21/2  "<HLSDem_KpNegHiCurr_mp>"
  cmp_21/1 -> Bitwise_And21/1
  Bitwise_And21/1 -> AndN/21, Scope/21, tws_21/1
  BS_Req/22 -> cmp_22/1, Scope22/1  "<testSig_HLSDem_PWinPosHiCurr_mp>"
  BS_Result/22 -> cmp_22/2, Scope22/2  "<HLSDem_PWinPosHiCurr_mp>"
  cmp_22/1 -> Bitwise_And22/1
  Bitwise_And22/1 -> AndN/22, Scope/22, tws_22/1
  BS_Req/23 -> cmp_23/1, Scope23/1  "<testSig_HLSDem_PWinNegHiCurr_mp>"
  BS_Result/23 -> cmp_23/2, Scope23/2  "<HLSDem_PWinNegHiCurr_mp>"
  cmp_23/1 -> Bitwise_And23/1
  Bitwise_And23/1 -> AndN/23, Scope/23, tws_23/1
  BS_Req/24 -> cmp_24/1, Scope24/1  "<testSig_HLSDem_KiHiCurr_mp>"
  BS_Result/24 -> cmp_24/2, Scope24/2  "<HLSDem_KiHiCurr_mp>"
  cmp_24/1 -> Bitwise_And24/1
  Bitwise_And24/1 -> AndN/24, Scope/24, tws_24/1
  BS_Req/25 -> cmp_25/1, Scope25/1  "<testSig_HLSDem_KiPosHiCurr_mp>"
  BS_Result/25 -> cmp_25/2, Scope25/2  "<HLSDem_KiPosHiCurr_mp>"
  cmp_25/1 -> Bitwise_And25/1
  Bitwise_And25/1 -> AndN/25, Scope/25, tws_25/1
  BS_Req/26 -> cmp_26/1, Scope26/1  "<testSig_HLSDem_KiNegHiCurr_mp>"
  BS_Result/26 -> cmp_26/2, Scope26/2  "<HLSDem_KiNegHiCurr_mp>"
  cmp_26/1 -> Bitwise_And26/1
  Bitwise_And26/1 -> AndN/26, Scope/26, tws_26/1
  BS_Req/27 -> cmp_27/1, Scope27/1  "<testSig_HLSDem_IWinPosHiCurr_mp>"
  BS_Result/27 -> cmp_27/2, Scope27/2  "<HLSDem_IWinPosHiCurr_mp>"
  cmp_27/1 -> Bitwise_And27/1
  Bitwise_And27/1 -> AndN/27, Scope/27, tws_27/1
  BS_Req/28 -> cmp_28/1, Scope28/1  "<testSig_HLSDem_IWinNegHiCurr_mp>"
  BS_Result/28 -> cmp_28/2, Scope28/2  "<HLSDem_IWinNegHiCurr_mp>"
  cmp_28/1 -> Bitwise_And28/1
  Bitwise_And28/1 -> AndN/28, Scope/28, tws_28/1

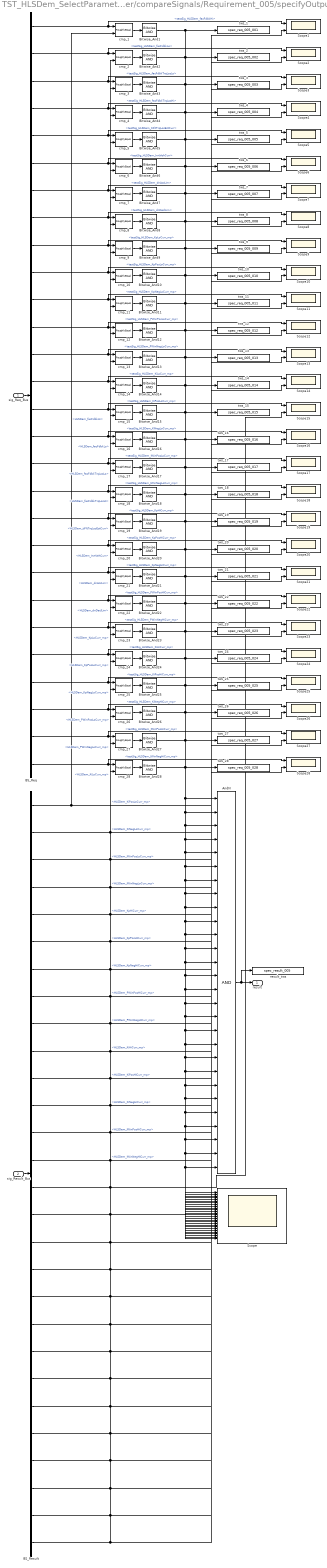
== system TST_HLSDem_SelectParameter/compareSignals/Requirement_005/specifyOutputs ==
  sig_Req_Bus : Inport
  sig_Result_Bus : Inport  Port=2
  AndN : Logic  Inputs=28
  BS_Req : BusSelector  OutputSignals=testSig_HLSDem_facFdbkHi,testSig_HLSDem_facFdbkLo,testSig_HLSDem_facFdbkTrqLosLo,testSig_HLSDem_facFdbkTrqLosHi,testSig_HLSDem_tiFltTrqLosEstCurr,testSig_HLSDem_InrtVehCurr,testSig_HLSDem_dnAccLim,testSig_HLSDem_dnDeclLim,testSig_HLSDem_KpLoCurr_mp,testSig_HLSDem_KpPosLoCurr_mp,testSig_HLSDem_KpNegLoCurr_mp,testSig_HLSDem_PWinPosLoCurr_mp,testSig_HLSDem_PWinNegLoCurr_mp,testSig_HLSDem_KiLoCurr_mp,testSig_HLSDem_KiPosLoCurr_mp,testSig_HLSDem_KiNegLoCurr_mp,testSig_HLSDem_IWinPosLoCurr_mp,testSig_HLSDem_IWinNegLoCurr_mp,testSig_HLSDem_KpHiCurr_mp,testSig_HLSDem_KpPosHiCurr_mp,testSig_HLSDem_KpNegHiCurr_mp,testSig_HLSDem_PWinPosHiCurr_mp,testSig_HLSDem_PWinNegHiCurr_mp,testSig_HLSDem_KiHiCurr_mp,testSig_HLSDem_KiPosHiCurr_mp,testSig_HLSDem_KiNegHiCurr_mp,testSig_HLSDem_IWinPosHiCurr_mp,testSig_HLSDem_IWinNegHiCurr_mp
  BS_Result : BusSelector  OutputSignals=HLSDem_facFdbkHi,HLSDem_facFdbkLo,HLSDem_facFdbkTrqLosLo,HLSDem_facFdbkTrqLosHi,HLSDem_tiFltTrqLosEstCurr,HLSDem_InrtVehCurr,HLSDem_dnAccLim,HLSDem_dnDeclLim,HLSDem_KpLoCurr_mp,HLSDem_KpPosLoCurr_mp,HLSDem_KpNegLoCurr_mp,HLSDem_PWinPosLoCurr_mp,HLSDem_PWinNegLoCurr_mp,HLSDem_KiLoCurr_mp,HLSDem_KiPosLoCurr_mp,HLSDem_KiNegLoCurr_mp,HLSDem_IWinPosLoCurr_mp,HLSDem_IWinNegLoCurr_mp,HLSDem_KpHiCurr_mp,HLSDem_KpPosHiCurr_mp,HLSDem_KpNegHiCurr_mp,HLSDem_PWinPosHiCurr_mp,HLSDem_PWinNegHiCurr_mp,HLSDem_KiHiCurr_mp,HLSDem_KiPosHiCurr_mp,HLSDem_KiNegHiCurr_mp,HLSDem_IWinPosHiCurr_mp,HLSDem_IWinNegHiCurr_mp
  Bitwise_And{1..28} (28 alike) : simulink/Logic and Bit Operations/Bitwise Operator  logicop=AND  UseBitMask=off  BitMask=bin2dec('11011001')  BitMaskRealWorld=Stored Integer
  Scope : Scope  NumInputPorts=28
  Scope{1..28} (28 alike) : Scope  NumInputPorts=2
  cmp_{1..6,9..28} (26 alike) : UnitTest_Lib/RoughlyEqual  slope=0.1
  cmp_7 : UnitTest_Lib/RoughlyEqual  slope=1
  cmp_8 : UnitTest_Lib/RoughlyEqual  slope=1
  result_tws : ToWorkspace  VariableName=spec_result_005
  tws_1 : ToWorkspace  VariableName=spec_req_005_001
  tws_10 : ToWorkspace  VariableName=spec_req_005_010
  tws_11 : ToWorkspace  VariableName=spec_req_005_011
  tws_12 : ToWorkspace  VariableName=spec_req_005_012
  tws_13 : ToWorkspace  VariableName=spec_req_005_013
  tws_14 : ToWorkspace  VariableName=spec_req_005_014
  tws_15 : ToWorkspace  VariableName=spec_req_005_015
  tws_16 : ToWorkspace  VariableName=spec_req_005_016
  tws_17 : ToWorkspace  VariableName=spec_req_005_017
  tws_18 : ToWorkspace  VariableName=spec_req_005_018
  tws_19 : ToWorkspace  VariableName=spec_req_005_019
  tws_2 : ToWorkspace  VariableName=spec_req_005_002
  tws_20 : ToWorkspace  VariableName=spec_req_005_020
  tws_21 : ToWorkspace  VariableName=spec_req_005_021
  tws_22 : ToWorkspace  VariableName=spec_req_005_022
  tws_23 : ToWorkspace  VariableName=spec_req_005_023
  tws_24 : ToWorkspace  VariableName=spec_req_005_024
  tws_25 : ToWorkspace  VariableName=spec_req_005_025
  tws_26 : ToWorkspace  VariableName=spec_req_005_026
  tws_27 : ToWorkspace  VariableName=spec_req_005_027
  tws_28 : ToWorkspace  VariableName=spec_req_005_028
  tws_3 : ToWorkspace  VariableName=spec_req_005_003
  tws_4 : ToWorkspace  VariableName=spec_req_005_004
  tws_5 : ToWorkspace  VariableName=spec_req_005_005
  tws_6 : ToWorkspace  VariableName=spec_req_005_006
  tws_7 : ToWorkspace  VariableName=spec_req_005_007
  tws_8 : ToWorkspace  VariableName=spec_req_005_008
  tws_9 : ToWorkspace  VariableName=spec_req_005_009
  result : Outport
  wires:
  sig_Req_Bus/1 -> BS_Req/1
  sig_Result_Bus/1 -> BS_Result/1
  AndN/1 -> result/1, result_tws/1
  BS_Req/1 -> cmp_1/1, Scope1/1  "<testSig_HLSDem_facFdbkHi>"
  BS_Result/1 -> cmp_1/2, Scope1/2  "<HLSDem_facFdbkHi>"
  cmp_1/1 -> Bitwise_And1/1
  Bitwise_And1/1 -> AndN/1, Scope/1, tws_1/1
  BS_Req/2 -> cmp_2/1, Scope2/1  "<testSig_HLSDem_facFdbkLo>"
  BS_Result/2 -> cmp_2/2, Scope2/2  "<HLSDem_facFdbkLo>"
  cmp_2/1 -> Bitwise_And2/1
  Bitwise_And2/1 -> AndN/2, Scope/2, tws_2/1
  BS_Req/3 -> cmp_3/1, Scope3/1  "<testSig_HLSDem_facFdbkTrqLosLo>"
  BS_Result/3 -> cmp_3/2, Scope3/2  "<HLSDem_facFdbkTrqLosLo>"
  cmp_3/1 -> Bitwise_And3/1
  Bitwise_And3/1 -> AndN/3, Scope/3, tws_3/1
  BS_Req/4 -> cmp_4/1, Scope4/1  "<testSig_HLSDem_facFdbkTrqLosHi>"
  BS_Result/4 -> cmp_4/2, Scope4/2  "<HLSDem_facFdbkTrqLosHi>"
  cmp_4/1 -> Bitwise_And4/1
  Bitwise_And4/1 -> AndN/4, Scope/4, tws_4/1
  BS_Req/5 -> cmp_5/1, Scope5/1  "<testSig_HLSDem_tiFltTrqLosEstCurr>"
  BS_Result/5 -> cmp_5/2, Scope5/2  "<HLSDem_tiFltTrqLosEstCurr>"
  cmp_5/1 -> Bitwise_And5/1
  Bitwise_And5/1 -> AndN/5, Scope/5, tws_5/1
  BS_Req/6 -> cmp_6/1, Scope6/1  "<testSig_HLSDem_InrtVehCurr>"
  BS_Result/6 -> cmp_6/2, Scope6/2  "<HLSDem_InrtVehCurr>"
  cmp_6/1 -> Bitwise_And6/1
  Bitwise_And6/1 -> AndN/6, Scope/6, tws_6/1
  BS_Req/7 -> cmp_7/1, Scope7/1  "<testSig_HLSDem_dnAccLim>"
  BS_Result/7 -> cmp_7/2, Scope7/2  "<HLSDem_dnAccLim>"
  cmp_7/1 -> Bitwise_And7/1
  Bitwise_And7/1 -> AndN/7, Scope/7, tws_7/1
  BS_Req/8 -> cmp_8/1, Scope8/1  "<testSig_HLSDem_dnDeclLim>"
  BS_Result/8 -> cmp_8/2, Scope8/2  "<HLSDem_dnDeclLim>"
  cmp_8/1 -> Bitwise_And8/1
  Bitwise_And8/1 -> AndN/8, Scope/8, tws_8/1
  BS_Req/9 -> cmp_9/1, Scope9/1  "<testSig_HLSDem_KpLoCurr_mp>"
  BS_Result/9 -> cmp_9/2, Scope9/2  "<HLSDem_KpLoCurr_mp>"
  cmp_9/1 -> Bitwise_And9/1
  Bitwise_And9/1 -> AndN/9, Scope/9, tws_9/1
  BS_Req/10 -> cmp_10/1, Scope10/1  "<testSig_HLSDem_KpPosLoCurr_mp>"
  BS_Result/10 -> cmp_10/2, Scope10/2  "<HLSDem_KpPosLoCurr_mp>"
  cmp_10/1 -> Bitwise_And10/1
  Bitwise_And10/1 -> AndN/10, Scope/10, tws_10/1
  BS_Req/11 -> cmp_11/1, Scope11/1  "<testSig_HLSDem_KpNegLoCurr_mp>"
  BS_Result/11 -> cmp_11/2, Scope11/2  "<HLSDem_KpNegLoCurr_mp>"
  cmp_11/1 -> Bitwise_And11/1
  Bitwise_And11/1 -> AndN/11, Scope/11, tws_11/1
  BS_Req/12 -> cmp_12/1, Scope12/1  "<testSig_HLSDem_PWinPosLoCurr_mp>"
  BS_Result/12 -> cmp_12/2, Scope12/2  "<HLSDem_PWinPosLoCurr_mp>"
  cmp_12/1 -> Bitwise_And12/1
  Bitwise_And12/1 -> AndN/12, Scope/12, tws_12/1
  BS_Req/13 -> cmp_13/1, Scope13/1  "<testSig_HLSDem_PWinNegLoCurr_mp>"
  BS_Result/13 -> cmp_13/2, Scope13/2  "<HLSDem_PWinNegLoCurr_mp>"
  cmp_13/1 -> Bitwise_And13/1
  Bitwise_And13/1 -> AndN/13, Scope/13, tws_13/1
  BS_Req/14 -> cmp_14/1, Scope14/1  "<testSig_HLSDem_KiLoCurr_mp>"
  BS_Result/14 -> cmp_14/2, Scope14/2  "<HLSDem_KiLoCurr_mp>"
  cmp_14/1 -> Bitwise_And14/1
  Bitwise_And14/1 -> AndN/14, Scope/14, tws_14/1
  BS_Req/15 -> cmp_15/1, Scope15/1  "<testSig_HLSDem_KiPosLoCurr_mp>"
  BS_Result/15 -> cmp_15/2, Scope15/2  "<HLSDem_KiPosLoCurr_mp>"
  cmp_15/1 -> Bitwise_And15/1
  Bitwise_And15/1 -> AndN/15, Scope/15, tws_15/1
  BS_Req/16 -> cmp_16/1, Scope16/1  "<testSig_HLSDem_KiNegLoCurr_mp>"
  BS_Result/16 -> cmp_16/2, Scope16/2  "<HLSDem_KiNegLoCurr_mp>"
  cmp_16/1 -> Bitwise_And16/1
  Bitwise_And16/1 -> AndN/16, Scope/16, tws_16/1
  BS_Req/17 -> cmp_17/1, Scope17/1  "<testSig_HLSDem_IWinPosLoCurr_mp>"
  BS_Result/17 -> cmp_17/2, Scope17/2  "<HLSDem_IWinPosLoCurr_mp>"
  cmp_17/1 -> Bitwise_And17/1
  Bitwise_And17/1 -> AndN/17, Scope/17, tws_17/1
  BS_Req/18 -> cmp_18/1, Scope18/1  "<testSig_HLSDem_IWinNegLoCurr_mp>"
  BS_Result/18 -> cmp_18/2, Scope18/2  "<HLSDem_IWinNegLoCurr_mp>"
  cmp_18/1 -> Bitwise_And18/1
  Bitwise_And18/1 -> AndN/18, Scope/18, tws_18/1
  BS_Req/19 -> cmp_19/1, Scope19/1  "<testSig_HLSDem_KpHiCurr_mp>"
  BS_Result/19 -> cmp_19/2, Scope19/2  "<HLSDem_KpHiCurr_mp>"
  cmp_19/1 -> Bitwise_And19/1
  Bitwise_And19/1 -> AndN/19, Scope/19, tws_19/1
  BS_Req/20 -> cmp_20/1, Scope20/1  "<testSig_HLSDem_KpPosHiCurr_mp>"
  BS_Result/20 -> cmp_20/2, Scope20/2  "<HLSDem_KpPosHiCurr_mp>"
  cmp_20/1 -> Bitwise_And20/1
  Bitwise_And20/1 -> AndN/20, Scope/20, tws_20/1
  BS_Req/21 -> cmp_21/1, Scope21/1  "<testSig_HLSDem_KpNegHiCurr_mp>"
  BS_Result/21 -> cmp_21/2, Scope21/2  "<HLSDem_KpNegHiCurr_mp>"
  cmp_21/1 -> Bitwise_And21/1
  Bitwise_And21/1 -> AndN/21, Scope/21, tws_21/1
  BS_Req/22 -> cmp_22/1, Scope22/1  "<testSig_HLSDem_PWinPosHiCurr_mp>"
  BS_Result/22 -> cmp_22/2, Scope22/2  "<HLSDem_PWinPosHiCurr_mp>"
  cmp_22/1 -> Bitwise_And22/1
  Bitwise_And22/1 -> AndN/22, Scope/22, tws_22/1
  BS_Req/23 -> cmp_23/1, Scope23/1  "<testSig_HLSDem_PWinNegHiCurr_mp>"
  BS_Result/23 -> cmp_23/2, Scope23/2  "<HLSDem_PWinNegHiCurr_mp>"
  cmp_23/1 -> Bitwise_And23/1
  Bitwise_And23/1 -> AndN/23, Scope/23, tws_23/1
  BS_Req/24 -> cmp_24/1, Scope24/1  "<testSig_HLSDem_KiHiCurr_mp>"
  BS_Result/24 -> cmp_24/2, Scope24/2  "<HLSDem_KiHiCurr_mp>"
  cmp_24/1 -> Bitwise_And24/1
  Bitwise_And24/1 -> AndN/24, Scope/24, tws_24/1
  BS_Req/25 -> cmp_25/1, Scope25/1  "<testSig_HLSDem_KiPosHiCurr_mp>"
  BS_Result/25 -> cmp_25/2, Scope25/2  "<HLSDem_KiPosHiCurr_mp>"
  cmp_25/1 -> Bitwise_And25/1
  Bitwise_And25/1 -> AndN/25, Scope/25, tws_25/1
  BS_Req/26 -> cmp_26/1, Scope26/1  "<testSig_HLSDem_KiNegHiCurr_mp>"
  BS_Result/26 -> cmp_26/2, Scope26/2  "<HLSDem_KiNegHiCurr_mp>"
  cmp_26/1 -> Bitwise_And26/1
  Bitwise_And26/1 -> AndN/26, Scope/26, tws_26/1
  BS_Req/27 -> cmp_27/1, Scope27/1  "<testSig_HLSDem_IWinPosHiCurr_mp>"
  BS_Result/27 -> cmp_27/2, Scope27/2  "<HLSDem_IWinPosHiCurr_mp>"
  cmp_27/1 -> Bitwise_And27/1
  Bitwise_And27/1 -> AndN/27, Scope/27, tws_27/1
  BS_Req/28 -> cmp_28/1, Scope28/1  "<testSig_HLSDem_IWinNegHiCurr_mp>"
  BS_Result/28 -> cmp_28/2, Scope28/2  "<HLSDem_IWinNegHiCurr_mp>"
  cmp_28/1 -> Bitwise_And28/1
  Bitwise_And28/1 -> AndN/28, Scope/28, tws_28/1
